simulink model "Modelo_simulink_masa_muelle_amortiguador"  (R2024a)
settings: Solver=VariableStepAuto  StartTime=0.0  StopTime=10.0  RelTol=1e-3
settings Model: Creator=BOUKA  LastModifiedBy=BOUKA

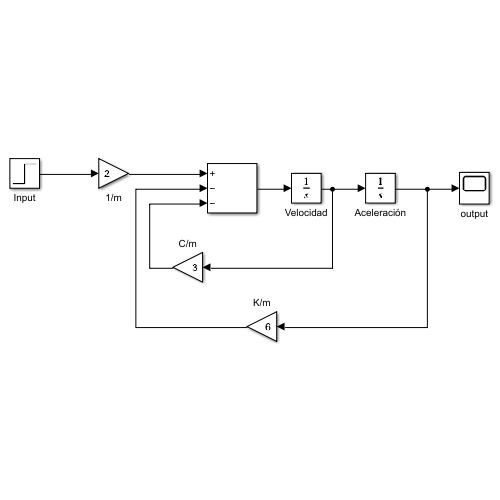
[thumbnail: Simulink's stored preview of the top-level diagram]
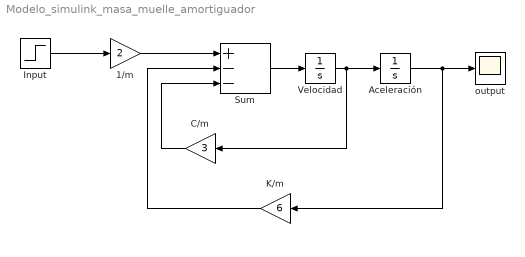
== system Modelo_simulink_masa_muelle_amortiguador ==
  1/m : Gain  Gain=2
  Aceleración : Integrator
  C/m : Gain  Gain=3
  Input : Step  Time=0  After=5  SampleTime=0
  K/m : Gain  Gain=6
  Sum : Sum  Inputs=+--
  Velocidad : Integrator  ContinuousStateAttributes='Velocidad'
  output : Scope
  wires:
  1/m/1 -> Sum/1
  C/m/1 -> Sum/3
  K/m/1 -> Sum/2
  Sum/1 -> Velocidad/1
  Velocidad/1 -> C/m/1, Aceleración/1
  Aceleración/1 -> K/m/1, output/1
  Input/1 -> 1/m/1
